simulink model "cell1D"  (R2014b)
settings: Solver=FixedStepDiscrete  StartTime=0.0  StopTime=100000  FixedStep=0.01  MaxStep=0.0001  RelTol=1e-3
settings Model: Creator=sand080  LastModifiedBy=sand080
settings DataIOCC: LimitDataPoints=off

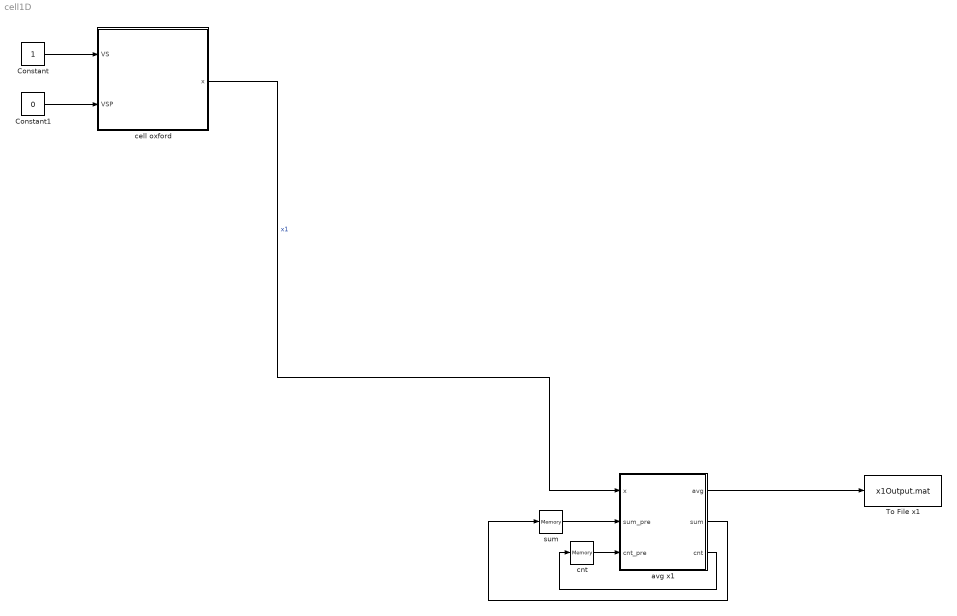
== system cell1D ==
  Constant : Constant
  Constant1 : Constant  Value=0
  To File x1 : ToFile  Filename=x1Output.mat
      settings: Decimation=10000000
  avg x1 : MATLAB Function  TreatAsAtomicUnit=on
  cell oxford : Subsystem
  cnt : Memory
  sum : Memory
  wires:
  cell oxford/1(x) -> avg x1/1(x)  "x1"
  avg x1/2(sum) -> sum/1
  avg x1/3(cnt) -> cnt/1
  cnt/1 -> avg x1/3(cnt_pre)
  sum/1 -> avg x1/2(sum_pre)
  avg x1/1(avg) -> To File x1/1
  Constant/1 -> cell oxford/1(VS)
  Constant1/1 -> cell oxford/2(VSP)

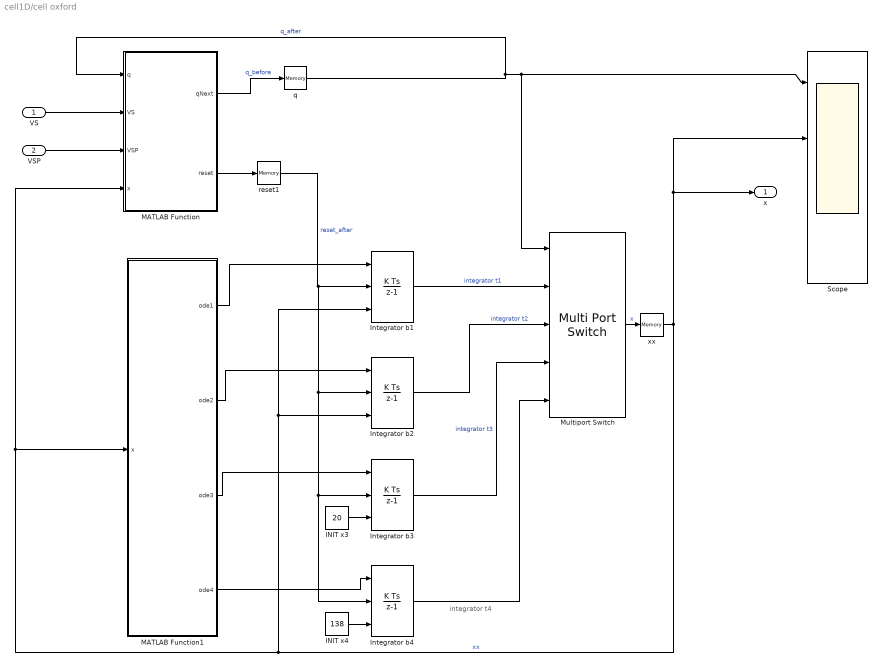
== system cell1D/cell oxford ==
  note: integrator t4
  VS : Inport
  VSP : Inport  Port=2
  INIT x3 : Constant  Value=20
  INIT x4 : Constant  Value=138
  Integrator b{1..4} (4 alike) : DiscreteIntegrator  ExternalReset=either  InitialConditionSource=external  InitialCondition=510  InitialConditionSetting=State (most efficient)  SampleTime=-1
  MATLAB Function : MATLAB Function  Priority=1  TreatAsAtomicUnit=on
  MATLAB Function1 : MATLAB Function  TreatAsAtomicUnit=on
  Multiport Switch : MultiPortSwitch  Inputs=4
  Scope : Scope  NumInputPorts=4
      settings: TickLabels=on  ShowLegends=on  YMin=0~0~0~0  YMax=1~1~1~1
  q : Memory  X0=1  LinearizeMemory=on
  reset1 : Memory  LinearizeMemory=on
  xx : Memory  X0=0.0001  LinearizeMemory=on
  x : Outport
  wires:
  xx/1 -> x/1, Scope/2, Integrator b1/3, Integrator b2/3, MATLAB Function1/1(x), MATLAB Function/4(x)  "xx"
  MATLAB Function1/1(ode1) -> Integrator b1/1
  MATLAB Function/1(qNext) -> q/1  "q_before"
  q/1 -> Scope/1, Multiport Switch/1, MATLAB Function/1(q)  "q_after"
  MATLAB Function/2(reset) -> reset1/1
  MATLAB Function1/2(ode2) -> Integrator b2/1
  INIT x3/1 -> Integrator b3/3
  MATLAB Function1/3(ode3) -> Integrator b3/1
  MATLAB Function1/4(ode4) -> Integrator b4/1
  reset1/1 -> Integrator b4/2, Integrator b3/2, Integrator b2/2, Integrator b1/2  "reset_after"
  Integrator b1/1 -> Multiport Switch/2  "integrator t1"
  Integrator b2/1 -> Multiport Switch/3  "integrator t2"
  Integrator b3/1 -> Multiport Switch/4  "integrator t3"
  Integrator b4/1 -> Multiport Switch/5
  VSP/1 -> MATLAB Function/3(VSP)
  VS/1 -> MATLAB Function/2(VS)
  Multiport Switch/1 -> xx/1  "x"
  INIT x4/1 -> Integrator b4/3

== matlab function cell1D/cell oxford/MATLAB Function ==
  data: q input; VS input; VSP input; x input; qNext output; reset output


function [qNext,reset]  = phi(q,  VS, VSP,x)
%#codegen


if q==1 % q=1, cell is resting
    if VS==0
        qNext=1;
        reset=0;
    elseif VS==1
        qNext=2;
        reset=1;
    else
        qNext=-1;
        reset=-1;
    end;
    
elseif q==2 % q=2, cell is stimulated
    if x<20 && VSP==1
        qNext=1;
        reset=1;
    elseif x< 20 && VSP==0
        qNext=2;
        reset=0;
    elseif x>= 20
        qNext=3;
        reset=1;
    else
        qNext=-1;
        reset=-1;
    end;

elseif q==3 % q=3, cell is upstroke
    if x >= 138
        qNext=4;
        reset=1;
    elseif x<138
        qNext=3;
        reset=0;
    else
        qNext=-1;
        reset=-1;
    end;
elseif q==4 % q=4, cell is plateau 
    if x<= 20
        qNext=1;
        reset=1;
    elseif x>20
        qNext=4;
        reset=0;
    else
        qNext=-1;
        reset=-1;
    end;
else
    qNext=-1; %this should never execute
    reset=-1;%this should never execute
end

== matlab function cell1D/cell oxford/MATLAB Function1 ==
  data: x input; ode1 output; ode2 output; ode3 output; ode4 output
function [ode1,ode2,ode3,ode4] = ODEs(x)
%#codegen

ode1=-0.1*x;
ode2=800;
ode3=200*x;
ode4=-0.002*x;

== matlab function cell1D/avg x1 ==
  data: x input; avg output; sum output; cnt output; sum_pre input; cnt_pre input
function [avg, sum,cnt] = fcn(x,  sum_pre, cnt_pre)
%#codegen

cnt=cnt_pre+1;
sum=sum_pre+x;
avg=sum/cnt;
